simulink model "Prob1"  (R2016b)
settings: Solver=ode1  StartTime=0.0  StopTime=10.0  RelTol=1e-3
values from neighbouring files (symbols this model uses):
  F_c = 1    [Prob1_par.m]
libraries: simulink x2
settings Model: Creator=helene  LastModifiedBy=helene

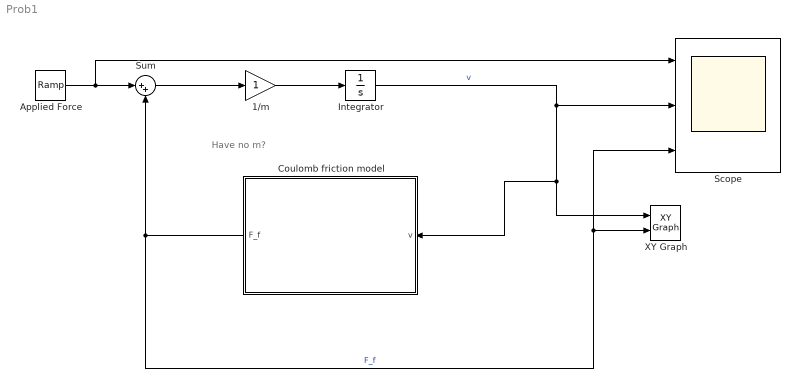
== system Prob1 ==
  note: Have no m?
  1/m : Gain
  "Applied Force " : simulink/Sources/Ramp  slope=0.5  start=0  X0=0
  Coulomb friction model : Subsystem
  Integrator : Integrator
  Scope : Scope  NumInputPorts=3
  Sum : Sum  Inputs=|++
  XY Graph : simulink/Sinks/XY Graph  xmin=-1  xmax=1  ymin=-1  ymax=1  st=-1
  wires:
  Sum/1 -> 1/m/1
  1/m/1 -> Integrator/1
  Coulomb friction model/1("F_f ") -> Sum/2, Scope/3, XY Graph/2  "F_f"
  Integrator/1 -> Scope/2, Coulomb friction model/1(v), XY Graph/1  "v"
  "Applied Force "/1 -> Scope/1, Sum/1

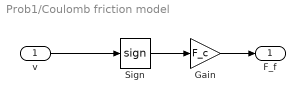
== system Prob1/Coulomb friction model ==
  v : Inport
  Gain : Gain  Gain=F_c
  Sign : Signum
  "F_f " : Outport
  wires:
  Sign/1 -> Gain/1
  v/1 -> Sign/1
  Gain/1 -> "F_f "/1
